simulink model "Maglev_Hardware_24a_R4"  (R2024a)
settings: Solver=FixedStepAuto  StartTime=0.0  StopTime=inf  FixedStep=.002  RelTol=1e-3  EnableMultiTasking=on
values from neighbouring files (symbols this model uses):
  cden = den{:}    [sim_maglev.m]
  cnum = num{:}    [sim_maglev.m]
undefined symbols (not defined in the file or in its folder): S
libraries: arduinolib x10, simulink x2
settings Model: ModifiedByFormat=C. Gokcek  SimulationMode=external  ExtModeTrigDuration=2  Creator=C. Gokcek  LastModifiedBy=C. Gokcek
settings SolverCC: AlgebraicLoopSolver=TrustRegion
settings DataIOCC: LimitDataPoints=on  SaveFormat=Array  ReturnWorkspaceOutputs=off
settings OptimizationCC: EnhancedBackFolding=on  PassReuseOutputArgsThreshold=0  MaxStackSize=64  OptimizeBlockOrder=speed  DifferentSizesBufferReuse=on  OptimizationCustomize=off
settings DebuggingCC: UnderspecifiedInitializationDetection=Classic  MergeDetectMultiDrivingBlocksExec=none  ParameterTunabilityLossMsg=error  UnconnectedInputMsg=warning  UnconnectedOutputMsg=warning  UnconnectedLineMsg=warning  StateNameClashWarn=warning  SFUnexpectedBacktrackingDiag=warning  SFNoUnconditionalDefaultTransitionDiag=warning  SFExecutionAtInitializationDiag=none  ArithmeticOperatorsInVariantConditions=warning
settings HardwareCC: ProdBitPerInt=16  ProdBitPerPointer=16  ProdBitPerSizeT=16  ProdBitPerPtrDiffT=16  ProdLargestAtomicFloat=None  ProdWordSize=8  ProdHWDeviceType=Atmel->AVR  UseEmbeddedCoderFeatures=off  UseSimulinkCoderFeatures=off
settings ModelReferenceCC: EnableRefExpFcnMdlSchedulingChecks=on  PropagateSignalLabelsOutOfModel=off
settings SFSimCC: SimUseLocalCustomCode=off  MATLABDynamicMemAlloc=off  CustomCodeUndefinedFunction=UseInterfaceOnly
settings RTWCC: Description=Embedded Coder  SystemTargetFile=ert.tlc  HardwareBoard=Arduino Mega 2560  TemplateMakefile=ert_default_tmf  RTWVerbose=off  RTWUseLocalCustomCode=off  Toolchain=Arduino AVR  BuildConfiguration=Faster Runs  GPUComputeCapability=3.5
settings CodeAppCC: ForceParamTrailComments=on  OperatorAnnotations=on  MangleLength=10
settings ERTTargetCC: ERTCustomFileBanners=off  SupportContinuousTime=on  SupportNonInlinedSFcns=on  RemoveResetFunc=off  SupportVariableSizeSignals=on  ModelStepFunctionPrototypeControlCompliant=off  ExtMode=on  ExtModeTransport=3  ExtModeStaticAlloc=on  ExtModeStaticAllocSize=2048  ExtModeMexFile=ext_xcp  ExtModeMexArgs=0 3 115200  ExtModeIntrfLevel=Level2 - Open  ERTSrcFileBannerTemplate=codertarget_code_template.cgt  ERTHdrFileBannerTemplate=codertarget_code_template.cgt  ERTDataSrcFileTemplate=codertarget_code_template.cgt  ERTDataHdrFileTemplate=codertarget_code_template.cgt
settings ConfigComp: CovMetricSettings=dw  CovSaveCumulativeToWorkspaceVar=on  CovSaveSingleToWorkspaceVar=on  CovExternalEMLEnable=off

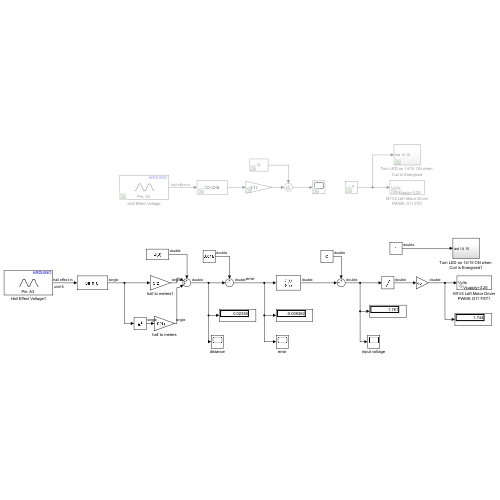
[thumbnail: Simulink's stored preview of the top-level diagram]
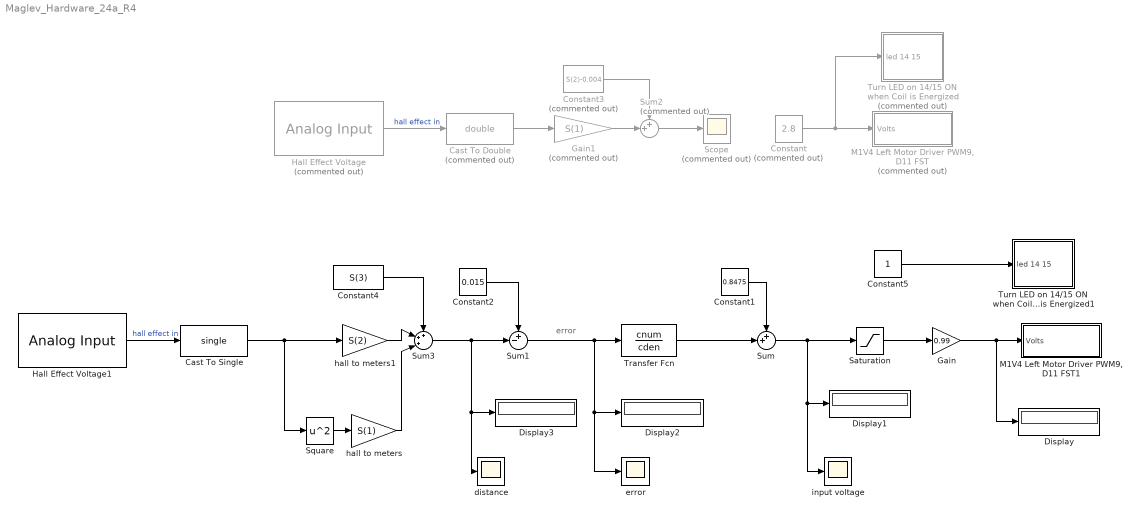
== system Maglev_Hardware_24a_R4 ==
  note: error
  Cast To Double : DataTypeConversion  Commented=on  OutDataTypeStr=double  SaturateOnIntegerOverflow=off  RndMeth=Floor
  Cast To Single : DataTypeConversion  OutDataTypeStr=single  SaturateOnIntegerOverflow=off  RndMeth=Floor
  Constant : Constant  Commented=on  Value=2.8
  Constant1 : Constant  Value=0.8475
  Constant2 : Constant  Value=0.015
  Constant3 : Constant  Commented=on  Value=S(2)-0.004
  Constant4 : Constant  Value=S(3)
  Constant5 : Constant
  Display{,1..3} (4 alike) : Display
  Gain : Gain  Gain=0.99
  Gain1 : Gain  Commented=on  Gain=S(1)
  Hall Effect Voltage : arduinolib/Analog Input  Commented=on  pinNumber=3  ReadResultsOnly=off  ConversionTriggerSource=Software  ExternalTriggerType=uint32( 0 )  OutputDataType=uint16  EnableConversionCompleteNotify=off  EnableOuputStatus=off  SampleTime=-1  blockPlatform=arduino
  Hall Effect Voltage1 : arduinolib/Analog Input  pinNumber=3  ReadResultsOnly=off  ConversionTriggerSource=Software  ExternalTriggerType=uint32( 0 )  OutputDataType=uint16  EnableConversionCompleteNotify=off  EnableOuputStatus=off  SampleTime=0.002  blockPlatform=arduino
  "M1V4 Left Motor Driver PWM9, D11 FST" : Subsystem  Commented=on  mask(Motor Driver){Vsupply=3.25}
      mask prompts: Vsupply "Driver Voltage"
      mask help:
      | Use a single PWM and a single Digtial out to control the magnitude and direction of a motor
      |
      | Specify driver supply voltage (3.25 for USB with SN754410)
      |
      | Driver supply voltage can be measured direcly by turning the motor fully on (100% duty cycle) and measuring the voltage across the motor leads.  This is the maximum voltage available to the motor and is used to scale from volts to PWM value 0-255.
      |
      | Note this value must be changed if the supply voltage to the driver is changed, for example, by using batteries.
      |
      | Vsupply is the maximum voltage your system is capable of supplying to system given the power supply. It needs to be measured depending on the power supply.
      mask Display:
      | port_label('input',1,'Volts')
      | text(15,5,['Vsupply=' num2str(Vsupply)])
  "M1V4 Left Motor Driver PWM9, D11 FST1" : Subsystem  mask(Motor Driver){Vsupply=3.25}
      mask prompts: Vsupply "Driver Voltage"
      mask help:
      | Use a single PWM and a single Digtial out to control the magnitude and direction of a motor
      |
      | Specify driver supply voltage (3.25 for USB with SN754410)
      |
      | Driver supply voltage can be measured direcly by turning the motor fully on (100% duty cycle) and measuring the voltage across the motor leads.  This is the maximum voltage available to the motor and is used to scale from volts to PWM value 0-255.
      |
      | Note this value must be changed if the supply voltage to the driver is changed, for example, by using batteries.
      |
      | Vsupply is the maximum voltage your system is capable of supplying to system given the power supply. It needs to be measured depending on the power supply.
      mask Display:
      | port_label('input',1,'Volts')
      | text(15,5,['Vsupply=' num2str(Vsupply)])
  Saturation : Saturate  UpperLimit=3.25  LowerLimit=-3.25
  Scope : Scope  Commented=on
  Square : Math  Operator=square
  Sum : Sum  Inputs=++|
  Sum1 : Sum  Inputs=+-|
  Sum2 : Sum  Commented=on  Inputs=++|
  Sum3 : Sum  Inputs=+++|
  Transfer Fcn : TransferFcn  Numerator=cnum  Denominator=cden
  Turn LED on 14/15 ON when Coil is Energized : Subsystem  Commented=on
  Turn LED on 14/15 ON when Coil is Energized1 : Subsystem
  distance : Scope
  error : Scope
  hall to meters : Gain  Gain=S(1)
  hall to meters1 : Gain  Gain=S(2)
  input voltage : Scope
  wires:
  Hall Effect Voltage/1 -> Cast To Double/1  "hall effect in"
  Constant/1 -> "M1V4 Left Motor Driver PWM9, D11 FST"/1(Volts), Turn LED on 14/15 ON when Coil is Energized/1(led 14 15)
  Hall Effect Voltage1/1 -> Cast To Single/1  "hall effect in"
  Constant1/1 -> Sum/1
  Constant2/1 -> Sum1/1
  Gain1/1 -> Sum2/2
  Sum2/1 -> Scope/1
  Constant3/1 -> Sum2/1
  Cast To Double/1 -> Gain1/1
  Sum3/1 -> Display3/1, distance/1, Sum1/2
  Constant4/1 -> Sum3/1
  Cast To Single/1 -> hall to meters1/1, Square/1
  Sum1/1 -> Transfer Fcn/1, error/1, Display2/1
  Transfer Fcn/1 -> Sum/2
  Sum/1 -> Display1/1, input voltage/1, Saturation/1
  Saturation/1 -> Gain/1
  hall to meters1/1 -> Sum3/2
  hall to meters/1 -> Sum3/3
  Square/1 -> hall to meters/1
  Gain/1 -> Display/1, "M1V4 Left Motor Driver PWM9, D11 FST1"/1(Volts)
  Constant5/1 -> Turn LED on 14/15 ON when Coil is Energized1/1(led 14 15)

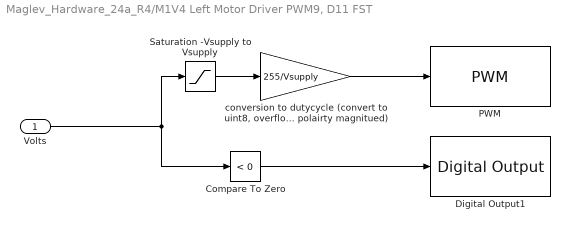
== system Maglev_Hardware_24a_R4/M1V4 Left Motor Driver PWM9, D11 FST ==
  Volts : Inport
  Compare To Zero : simulink/Logic and Bit Operations/Compare To Zero  relop=<  OutDataTypeStr=boolean
  Digital Output1 : arduinolib/Digital Output  pinNumber=11  Direction=output  blockPlatform=arduino
  PWM : arduinolib/PWM  pinNumber=9  frequencyType=Default  desiredFrequency=490.2  achievableFrequency=490.2
  Saturation -Vsupply to Vsupply : Saturate  UpperLimit=Vsupply  LowerLimit=-Vsupply  OutDataTypeStr=single
  "conversion to dutycycle (convert to uint8, overflow will provide reverse polairty magnitued)" : Gain  Gain=255/Vsupply  OutDataTypeStr=uint8
  wires:
  Volts/1 -> Compare To Zero/1, Saturation -Vsupply to Vsupply/1
  Saturation -Vsupply to Vsupply/1 -> "conversion to dutycycle (convert to uint8, overflow will provide reverse polairty magnitued)"/1
  "conversion to dutycycle (convert to uint8, overflow will provide reverse polairty magnitued)"/1 -> PWM/1
  Compare To Zero/1 -> Digital Output1/1

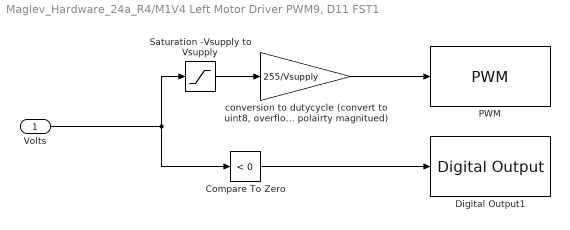
== system Maglev_Hardware_24a_R4/M1V4 Left Motor Driver PWM9, D11 FST1 ==
  Volts : Inport
  Compare To Zero : simulink/Logic and Bit Operations/Compare To Zero  relop=<  OutDataTypeStr=boolean
  Digital Output1 : arduinolib/Digital Output  pinNumber=11  Direction=output  blockPlatform=arduino
  PWM : arduinolib/PWM  pinNumber=9  frequencyType=Default  desiredFrequency=490.2  achievableFrequency=490.2
  Saturation -Vsupply to Vsupply : Saturate  UpperLimit=Vsupply  LowerLimit=-Vsupply  OutDataTypeStr=single
  "conversion to dutycycle (convert to uint8, overflow will provide reverse polairty magnitued)" : Gain  Gain=255/Vsupply  OutDataTypeStr=uint8
  wires:
  Volts/1 -> Compare To Zero/1, Saturation -Vsupply to Vsupply/1
  Saturation -Vsupply to Vsupply/1 -> "conversion to dutycycle (convert to uint8, overflow will provide reverse polairty magnitued)"/1
  "conversion to dutycycle (convert to uint8, overflow will provide reverse polairty magnitued)"/1 -> PWM/1
  Compare To Zero/1 -> Digital Output1/1

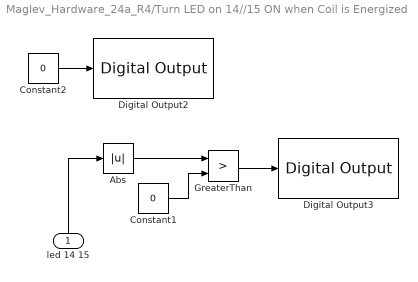
== system Maglev_Hardware_24a_R4/Turn LED on 14//15 ON when Coil is Energized ==
  led 14 15 : Inport
  Abs : Abs  SaturateOnIntegerOverflow=off
  Constant1 : Constant  Value=0  OutDataTypeStr=boolean  SampleTime=0
  Constant2 : Constant  Value=0  OutDataTypeStr=boolean  SampleTime=0
  Digital Output2 : arduinolib/Digital Output  pinNumber=14  Direction=output  blockPlatform=arduino
  Digital Output3 : arduinolib/Digital Output  pinNumber=15  Direction=output  blockPlatform=arduino
  GreaterThan : RelationalOperator  Operator=>  OutDataTypeStr=boolean  RndMeth=Simplest  InputSameDT=off
  wires:
  Constant2/1 -> Digital Output2/1
  led 14 15/1 -> Abs/1
  Abs/1 -> GreaterThan/1
  Constant1/1 -> GreaterThan/2
  GreaterThan/1 -> Digital Output3/1

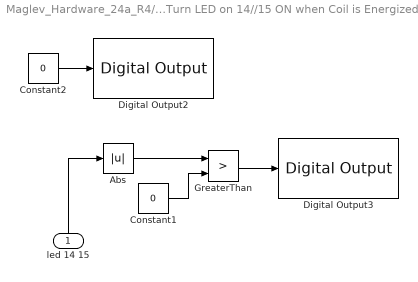
== system Maglev_Hardware_24a_R4/Turn LED on 14//15 ON when Coil is Energized1 ==
  led 14 15 : Inport
  Abs : Abs  SaturateOnIntegerOverflow=off
  Constant1 : Constant  Value=0  OutDataTypeStr=boolean  SampleTime=0
  Constant2 : Constant  Value=0  OutDataTypeStr=boolean  SampleTime=0
  Digital Output2 : arduinolib/Digital Output  pinNumber=14  Direction=output  blockPlatform=arduino
  Digital Output3 : arduinolib/Digital Output  pinNumber=15  Direction=output  blockPlatform=arduino
  GreaterThan : RelationalOperator  Operator=>  OutDataTypeStr=boolean  RndMeth=Simplest  InputSameDT=off
  wires:
  Constant2/1 -> Digital Output2/1
  led 14 15/1 -> Abs/1
  Abs/1 -> GreaterThan/1
  Constant1/1 -> GreaterThan/2
  GreaterThan/1 -> Digital Output3/1
